simulink model "building_EXAMPLE_v1"  (R2016b)
settings: Solver=ode23tb  StartTime=-building.preruntime+8760*3600  StopTime=building.runtime+8760*3600  MaxStep=600  EnableMultiTasking=on
StartFcn:
  | tic
StopFcn:
  | toc
values from neighbouring files (symbols this model uses):
  building = create_building_automatic(building, modify, import_mode, name_XML, name_EXCEL, name_PHPP, NUMBEROFZONES)    [work_EXAMPLE_v1.m]
undefined symbols (not defined in the file or in its folder): A, B, C, cp, Dd, Dreifach, FluidMix, get_building, ID, MassFlow, p, Pressure, Qdot_C, Qdot_C_energy, Qdot_H, Qdot_H_energy, Qdot_I_electricity, Qdot_I_electricity_energy, Qdot_I_light, Qdot_I_light_energy, Qdot_I_person, Qdot_I_person_energy, Qdot_S, Qdot_S_energy, Qdot_T_ground, Qdot_T_ground_energy, Qdot_T_neighbour, Qdot_T_neighbour_energy, Qdot_T_opaque, Qdot_T_opaque_energy, Qdot_T_window, Qdot_T_window_energy, Qdot_V_infiltration, Qdot_V_infiltration_energy, Qdot_V_mech, Qdot_V_mech_energy, Qdot_V_window, Qdot_V_window_energy, rho, Tc, Temperature, Tr, Ts, Wärmeschutzglas, x_CO2, x_H2O, x_VOC
libraries: carnotUIBK x1931, carnot x83, simulink_extras x22, simulink x12
(part 3 of 35)

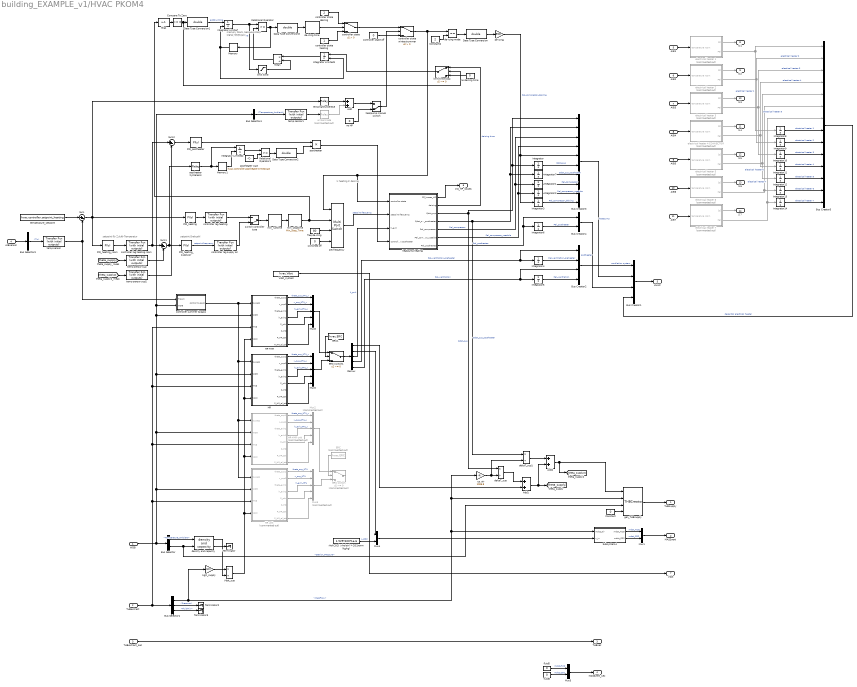
== system building_EXAMPLE_v1/HVAC PKOM4 ==
  note: setpoint Drehzahl
  note: setpoint für Zuluft-Temperatur
  note: memory block,
      | because sharp
      | signal necessary
  note: 1: heating
      | 2: deicing
  WDB : Inport
  THBextract : Inport  Port=2
  THBextract_sec : Inport  Port=3
  AIBsensor : Inport  Port=4
  AIB1 : Inport  Port=5
  AIB2 : Inport  Port=6
  AIB3 : Inport  Port=7
  AIB4 : Inport  Port=8
  AIB5 : Inport  Port=9
  AIB6 : Inport  Port=10
  AIB7 : Inport  Port=11
  Add : Sum
  Add1 : Sum
  Add2 : Sum
  Bias : Bias  Bias=-1
  Bus Creator1 : BusCreator  Inputs=4
  Bus Creator2 : BusCreator  Inputs=4
  Bus Creator3 : BusCreator  Inputs=10
  Bus Creator4 : BusCreator  Inputs=2
  Bus Creator5 : BusCreator  Inputs=14
  Bus Selector : BusSelector  OutputSignals=Temperature_Ambient,Station_Pressure
  Bus Selector1 : BusSelector  OutputSignals=MassFlow,Pressure,FluidMix
  Bus Selector3 : BusSelector  OutputSignals=Ts
  Bus Selector4 : BusSelector  OutputSignals=Temperature_Ambient
  Compare To Zero : simulink/Logic and Bit Operations/Compare To Zero  relop=>=  OutDataTypeStr=uint8
  Constant : Constant  Value=0
  Constant2 : Constant  Value=2
  Data Type Conversion{,1..3} (4 alike) : DataTypeConversion  OutDataTypeStr=double
  Demux : Demux  Outputs=5
  ERC : Constant  Commented=on  Value=hvac.ERC
  ERC switch : Switch  Commented=on  Criteria=u2 ~= 0
  ERC switch1 : Switch  Criteria=u2 ~= 0
  ERC1 : Constant  Value=hvac.ERC
  Einschalthysterese : Relay  OnSwitchValue=0.5  OffSwitchValue=-0.5
  HR : Subsystem  mask{p_el=hvac.HRC_NTU_lu.p_el, low_lim=hvac.HRC_NTU_lu.preheater, Vdot=hvac.HRC_NTU_lu.Vdot, NTU=hvac.HRC_NTU_lu.NTU, NTU_x=hvac.HRC_NTU_lu.NTU_x, vent_sup=off, vent_ext=on, vent_amb=on, vent_exh=off}
      mask prompts: p_el "specific ventilator power in [Wh/m^3]"; low_lim "ambient temperature at which pre-heater starts"; Vdot "volume flow in [m^3/h] for NTU"; NTU_x "NTU of moisture recovery"; vent_sup "ventilator in supply air"; vent_ext "ventilator in extract air"; vent_amb "ventilator in ambient air"; vent_exh "ventilator in exhaust air"
  HR unit : Subsystem  Commented=on  mask{theta_amb2=hvac.HRC_NTU(hvac.system).theta_amb, theta_ext1=hvac.HRC_NTU(hvac.system).theta_ext, Vdot=hvac.HRC_NTU(hvac.system).Vdot, P_el=hvac.HRC_NTU(hvac.system).p_el, rec=hvac.HRC_NTU(hvac.system).eta_phi, low_lim=hvac.HRC_NTU(hvac.system).preheater, vent_sup=off, vent_exh=off, vent_amb=on, vent_ext=on}
      mask prompts: theta_amb2 "ambient air temperature for NTU calculation"; theta_ext1 "extract air temperature for NTU calculation"; Vdot "volume flow in [m^3/h] for NTU"; P_el "specific ventilator power in [Wh/m^3]"; rec "efficiency of heat recovery (by PHI)"; low_lim "ambient temperature at which pre-heater starts"; vent_sup "ventilator in supply air"; vent_exh "ventilator in exhaust air"; vent_amb "ventilator in ambient air"; vent_ext "ventilator in extract air"
      mask init:
      | cp_a = heat_capacity(theta_ext1,1E5,2,0);
      | rho_a = density(theta_ext1,1E5,2,0);
      | mdot_cp = Vdot * cp_a * rho_a / 3600;
      | 
      | %%% NTU %%
      | % not humidity (condensation) considered
      | P_elec = P_el * Vdot;
      | 
      | theta_amb1 = theta_amb2;
      | theta_amb0 = theta_amb1 + vent_amb * P_elec/mdot_cp/2;
      | theta_ext0 = theta_ext1 + vent_ext * P_elec/mdot_cp/2;
      | theta_exh1 = theta_ext1 + P_elec/mdot_cp - rec * (theta_ext1 - theta_amb1);
      | theta_exh0 = theta_exh1 - vent_exh * P_elec/mdot_cp/2;
      | theta_sup0 = theta_amb0 + theta_ext0 - theta_exh0;
      | theta_sup1 = theta_sup0 + vent_sup * P_elec/mdot_cp/2;
      | 
      | dtheta_log = (theta_exh0-theta_amb0 + theta_ext0-theta_sup0)/2;
      | 
      | P_HX = mdot_cp * (theta_sup0-theta_amb1);
      | UA = P_HX / dtheta_log;
      | NTU = UA / mdot_cp;
      | 
      | disp(['  NTU = ' num2str(NTU)])
  HR+MR : Subsystem  mask{p_el=hvac.ERC_NTU_lu.p_el, low_lim=hvac.ERC_NTU_lu.preheater, Vdot=hvac.ERC_NTU_lu.Vdot, NTU=hvac.ERC_NTU_lu.NTU, NTU_x=hvac.ERC_NTU_lu.NTU_x, vent_sup=off, vent_ext=on, vent_amb=on, vent_exh=off}
      mask prompts: p_el "specific ventilator power in [Wh/m^3]"; low_lim "ambient temperature at which pre-heater starts"; Vdot "volume flow in [m^3/h] for NTU"; NTU_x "NTU of moisture recovery"; vent_sup "ventilator in supply air"; vent_ext "ventilator in extract air"; vent_amb "ventilator in ambient air"; vent_exh "ventilator in exhaust air"
  HR+MR unit : Subsystem  Commented=on  mask{theta_amb2=hvac.ERC_NTU(hvac.system).theta_amb, theta_ext1=hvac.ERC_NTU(hvac.system).theta_ext, Vdot=hvac.ERC_NTU(hvac.system).Vdot, P_el=hvac.ERC_NTU(hvac.system).p_el, rec=hvac.ERC_NTU(hvac.system).eta_phi, low_lim=hvac.ERC_NTU(hvac.system).preheater, NTU_x=hvac.ERC_NTU(hvac.system).NTU_x, vent_sup=off, vent_exh=off, vent_amb=on, vent_ext=on}
      mask prompts: theta_amb2 "ambient air temperature for NTU calculation"; theta_ext1 "extract air temperature for NTU calculation"; Vdot "volume flow in [m^3/h] for NTU"; P_el "specific ventilator power in [Wh/m^3]"; rec "efficiency of heat recovery (by PHI)"; low_lim "ambient temperature at which pre-heater starts"; NTU_x "NTU of moisture recovery"; vent_sup "ventilator in supply air"; vent_exh "ventilator in exhaust air"; vent_amb "ventilator in ambient air"; vent_ext "ventilator in extract air"
      mask init:
      | cp_a = heat_capacity(theta_ext1,1E5,2,0);
      | rho_a = density(theta_ext1,1E5,2,0);
      | mdot_cp = Vdot * cp_a * rho_a / 3600;
      | 
      | %%% NTU %%
      | % not humidity (condensation) considered
      | P_elec = P_el * Vdot;
      | 
      | theta_amb1 = theta_amb2;
      | theta_amb0 = theta_amb1 + vent_amb * P_elec/mdot_cp/2;
      | theta_ext0 = theta_ext1 + vent_ext * P_elec/mdot_cp/2;
      | theta_exh1 = theta_ext1 + P_elec/mdot_cp - rec * (theta_ext1 - theta_amb1);
      | theta_exh0 = theta_exh1 - vent_exh * P_elec/mdot_cp/2;
      | theta_sup0 = theta_amb0 + theta_ext0 - theta_exh0;
      | theta_sup1 = theta_sup0 + vent_sup * P_elec/mdot_cp/2;
      | 
      | dtheta_log = (theta_exh0-theta_amb0 + theta_ext0-theta_sup0)/2;
      | 
      | P_HX = mdot_cp * (theta_sup0-theta_amb1);
      | UA = P_HX / dtheta_log;
      | NTU = UA / mdot_cp;
      | 
      | disp(['  NTU = ' num2str(NTU)])
      | disp(['  NTU_x = ' num2str(NTU_x)])
  Integrator{,1..14} (15 alike) : Integrator
  Integrator Limited : Integrator  ExternalReset=rising  LimitOutput=on  LowerSaturationLimit=0
  Integrator Limited1 : Integrator  ExternalReset=rising  LimitOutput=on  LowerSaturationLimit=0
  Integrator Limited2 : Integrator  ExternalReset=either  LimitOutput=on  LowerSaturationLimit=0
  Memory : Memory
  Memory1 : Memory
  Mux1 : Mux  Inputs=2
  Mux2 : Mux  Commented=on  Inputs=5
  Mux3 : Mux  Inputs=2
  Mux4 : Mux  Inputs=2
  Mux5 : Mux  Commented=on  Inputs=5
  Mux6 : Mux  Inputs=5
  Mux8 : Mux  Inputs=5
  PID_heating : simulink/Continuous/PID Controller  Controller=PI  TimeDomain=Continuous-time  SampleTime=-1  IntegratorMethod=Forward Euler  FilterMethod=Forward Euler  Form=Ideal  UseFilter=on  ControllerParametersSource=internal  P=2  I=0.01  D=0  N=100  InitialConditionSource=internal  InitialConditionForIntegrator=0  InitialConditionForFilter=0  ExternalReset=none  LimitOutput=on  UpperSaturationLimit=80  LowerSaturationLimit=0  LinearizeAsGain=on  AntiWindupMode=clamping  Kb=1  TrackingMode=off  Kt=1  PParamMin=[]  PParamMax=[]  IParamMin=[]  IParamMax=[]  DParamMin=[]  DParamMax=[]  NParamMin=[]  NParamMax=[]  KbParamMin=[]  KbParamMax=[]  KtParamMin=[]  KtParamMax=[]  POutMin=[]  POutMax=[]  IOutMin=[]  IOutMax=[]  DOutMin=[]  DOutMax=[]  NOutMin=[]  NOutMax=[]  KbOutMin=[]  KbOutMax=[]  KtOutMin=[]  KtOutMax=[]  IntegratorOutMin=[]  IntegratorOutMax=[]  FilterOutMin=[]  FilterOutMax=[]  SumOutMin=[]  SumOutMax=[]  SumI1OutMin=[]  SumI1OutMax=[]  SumI2OutMin=[]  SumI2OutMax=[]  SumI3OutMin=[]  SumI3OutMax=[]  SumDOutMin=[]  SumDOutMax=[]  SaturationOutMin=[]  SaturationOutMax=[]  IntegratorContinuousStateAttributes=''  IntegratorStateMustResolveToSignalObject=off  IntegratorRTWStateStorageClass=Auto  FilterContinuousStateAttributes=''  FilterStateMustResolveToSignalObject=off  FilterRTWStateStorageClass=Auto  DifferentiatorICPrevScaledInput=0  DifferentiatorOutMin=[]  DifferentiatorOutMax=[]
  PID_heating_room : simulink/Continuous/PID Controller  Controller=PI  TimeDomain=Continuous-time  SampleTime=-1  IntegratorMethod=Forward Euler  FilterMethod=Forward Euler  Form=Ideal  UseFilter=on  ControllerParametersSource=internal  P=hvac.controller.PID_heating_room.P  I=hvac.controller.PID_heating_room.I  D=0  N=100  InitialConditionSource=internal  InitialConditionForIntegrator=0  InitialConditionForFilter=0  ExternalReset=none  LimitOutput=on  UpperSaturationLimit=hvac.controller.PID_heating_room.upper_limit  LowerSaturationLimit=hvac.controller.PID_heating_room.lower_limit  LinearizeAsGain=on  AntiWindupMode=clamping  Kb=1  TrackingMode=off  Kt=1  PParamMin=[]  PParamMax=[]  IParamMin=[]  IParamMax=[]  DParamMin=[]  DParamMax=[]  NParamMin=[]  NParamMax=[]  KbParamMin=[]  KbParamMax=[]  KtParamMin=[]  KtParamMax=[]  POutMin=[]  POutMax=[]  IOutMin=[]  IOutMax=[]  DOutMin=[]  DOutMax=[]  NOutMin=[]  NOutMax=[]  KbOutMin=[]  KbOutMax=[]  KtOutMin=[]  KtOutMax=[]  IntegratorOutMin=[]  IntegratorOutMax=[]  FilterOutMin=[]  FilterOutMax=[]  SumOutMin=[]  SumOutMax=[]  SumI1OutMin=[]  SumI1OutMax=[]  SumI2OutMin=[]  SumI2OutMax=[]  SumI3OutMin=[]  SumI3OutMax=[]  SumDOutMin=[]  SumDOutMax=[]  SaturationOutMin=[]  SaturationOutMax=[]  IntegratorContinuousStateAttributes=''  IntegratorStateMustResolveToSignalObject=off  IntegratorRTWStateStorageClass=Auto  FilterContinuousStateAttributes=''  FilterStateMustResolveToSignalObject=off  FilterRTWStateStorageClass=Auto  DifferentiatorICPrevScaledInput=0  DifferentiatorOutMin=[]  DifferentiatorOutMax=[]
  PID_heating_supplyair : simulink/Continuous/PID Controller  Controller=PI  TimeDomain=Continuous-time  SampleTime=-1  IntegratorMethod=Forward Euler  FilterMethod=Forward Euler  Form=Ideal  UseFilter=on  ControllerParametersSource=internal  P=hvac.controller.PID_heating_supplyair.P  I=hvac.controller.PID_heating_supplyair.I  D=0  N=100  InitialConditionSource=internal  InitialConditionForIntegrator=0  InitialConditionForFilter=0  ExternalReset=none  LimitOutput=on  UpperSaturationLimit=hvac.controller.PID_heating_supplyair.upper_limit  LowerSaturationLimit=hvac.controller.PID_heating_supplyair.lower_limit  LinearizeAsGain=on  AntiWindupMode=clamping  Kb=1  TrackingMode=off  Kt=1  PParamMin=[]  PParamMax=[]  IParamMin=[]  IParamMax=[]  DParamMin=[]  DParamMax=[]  NParamMin=[]  NParamMax=[]  KbParamMin=[]  KbParamMax=[]  KtParamMin=[]  KtParamMax=[]  POutMin=[]  POutMax=[]  IOutMin=[]  IOutMax=[]  DOutMin=[]  DOutMax=[]  NOutMin=[]  NOutMax=[]  KbOutMin=[]  KbOutMax=[]  KtOutMin=[]  KtOutMax=[]  IntegratorOutMin=[]  IntegratorOutMax=[]  FilterOutMin=[]  FilterOutMax=[]  SumOutMin=[]  SumOutMax=[]  SumI1OutMin=[]  SumI1OutMax=[]  SumI2OutMin=[]  SumI2OutMax=[]  SumI3OutMin=[]  SumI3OutMax=[]  SumDOutMin=[]  SumDOutMax=[]  SaturationOutMin=[]  SaturationOutMax=[]  IntegratorContinuousStateAttributes=''  IntegratorStateMustResolveToSignalObject=off  IntegratorRTWStateStorageClass=Auto  FilterContinuousStateAttributes=''  FilterStateMustResolveToSignalObject=off  FilterRTWStateStorageClass=Auto  DifferentiatorICPrevScaledInput=0  DifferentiatorOutMin=[]  DifferentiatorOutMax=[]
  PID_postheater : simulink/Continuous/PID Controller  Controller=PI  TimeDomain=Continuous-time  SampleTime=-1  IntegratorMethod=Forward Euler  FilterMethod=Forward Euler  Form=Ideal  UseFilter=on  ControllerParametersSource=internal  P=hvac.controller.postheater.PID.P  I=hvac.controller.postheater.PID.I  D=0  N=100  InitialConditionSource=internal  InitialConditionForIntegrator=0  InitialConditionForFilter=0  ExternalReset=none  LimitOutput=on  UpperSaturationLimit=hvac.controller.postheater.PID.upper_limit  LowerSaturationLimit=hvac.controller.postheater.PID.lower_limit  LinearizeAsGain=on  AntiWindupMode=clamping  Kb=1  TrackingMode=off  Kt=1  PParamMin=[]  PParamMax=[]  IParamMin=[]  IParamMax=[]  DParamMin=[]  DParamMax=[]  NParamMin=[]  NParamMax=[]  KbParamMin=[]  KbParamMax=[]  KtParamMin=[]  KtParamMax=[]  POutMin=[]  POutMax=[]  IOutMin=[]  IOutMax=[]  DOutMin=[]  DOutMax=[]  NOutMin=[]  NOutMax=[]  KbOutMin=[]  KbOutMax=[]  KtOutMin=[]  KtOutMax=[]  IntegratorOutMin=[]  IntegratorOutMax=[]  FilterOutMin=[]  FilterOutMax=[]  SumOutMin=[]  SumOutMax=[]  SumI1OutMin=[]  SumI1OutMax=[]  SumI2OutMin=[]  SumI2OutMax=[]  SumI3OutMin=[]  SumI3OutMax=[]  SumDOutMin=[]  SumDOutMax=[]  SaturationOutMin=[]  SaturationOutMax=[]  IntegratorContinuousStateAttributes=''  IntegratorStateMustResolveToSignalObject=off  IntegratorRTWStateStorageClass=Auto  FilterContinuousStateAttributes=''  FilterStateMustResolveToSignalObject=off  FilterRTWStateStorageClass=Auto  DifferentiatorICPrevScaledInput=0  DifferentiatorOutMin=[]  DifferentiatorOutMax=[]
  Relational Operator : RelationalOperator  OutDataTypeStr=boolean  RndMeth=Simplest
  Relational Operator1 : RelationalOperator  OutDataTypeStr=boolean  RndMeth=Simplest
  Subsystem4 : Subsystem
  Sum : Sum  Inputs=|+-
  Sum1 : Sum  Inputs=|+-
  Sum2 : Sum  Inputs=|+-
  Terminator : Terminator
  Terminator2 : Terminator
  Terminator3 : Terminator
  Vdot_sup : Product  Inputs=*/
  Vdot_system : Constant  Value=hvac.Vdot
  controller lag heating : simulink_extras/Additional Linear/Transfer Fcn (with initial outputs)  N=[1]  D=[60 1]  Y0=20  U0=0
  controller lag heating room : simulink_extras/Additional Linear/Transfer Fcn (with initial outputs)  N=[1]  D=[60 1]  Y0=20  U0=0
  controller lag supply air : simulink_extras/Additional Linear/Transfer Fcn (with initial outputs)  N=[1]  D=[60 1]  Y0=20  U0=0
  controller state : Switch  Criteria=u2 > Threshold
  controller state deicing : Constant  Value=2
  controller state heating : Constant
  controller state off : Constant  Value=0
  controller state winter/summer : Switch  Criteria=u2 > Threshold
  controller summer bypass : Subsystem
  cp_air : Gain  Gain=1006.8
  de-icing : Gain  Gain=550
  de-icing mode : RelationalOperator  Operator===  OutDataTypeStr=boolean  RndMeth=Simplest
  de-icing time : carnot/Control/Min_Run_Time  tminrun=hvac.controller.deicing_time  mv=1
  deltaT_sup : Product  Inputs=*/
  deltaT_sup1 : Product  Inputs=*/
  density and capacity : carnotUIBK/general/density and capacity
  electrical heater 1 : Subsystem  Commented=on  mask{theta_r_t=hvac.controller.electricalheater.zone(1).theta_r_t, theta_r_t_low=hvac.controller.electricalheater.zone(1).theta_r_t_low, max_power=hvac.controller.electricalheater.zone(1).max_power, part_rad=hvac.controller.electricalheater.zone(1).part_rad, timeconstant_heater=hvac.controller.electricalheater.zone(1).timeconstant_heater, Kp=hvac.controller.electricalheater.zone(1).Kp, Tn=hvac.controller.electricalheater.zone(1).Tn, control_time_values=hvac.controller.electricalheater.zone(1).control_time_values, control_time_duration=hvac.controller.electricalheater.zone(1).control_time_duration, control_time_output=hvac.controller.electricalheater.zone(1).control_time_output}
      mask prompts: theta_r_t "setpoint"; theta_r_t_low "setpoint off/night"; max_power "maximal power"; part_rad "part of radiation"; timeconstant_heater "timeconstant heater"; Kp "PID Kp"; Tn "PID Tn"; control_time_values "control time values"; control_time_duration "control time duration"; control_time_output "control time output"
  electrical heater 2 : Subsystem  Commented=on  mask{theta_r_t=hvac.controller.electricalheater.zone(2).theta_r_t, theta_r_t_low=hvac.controller.electricalheater.zone(2).theta_r_t_low, max_power=hvac.controller.electricalheater.zone(2).max_power, part_rad=hvac.controller.electricalheater.zone(2).part_rad, timeconstant_heater=hvac.controller.electricalheater.zone(2).timeconstant_heater, Kp=hvac.controller.electricalheater.zone(2).Kp, Tn=hvac.controller.electricalheater.zone(2).Tn, control_time_values=hvac.controller.electricalheater.zone(2).control_time_values, control_time_duration=hvac.controller.electricalheater.zone(2).control_time_duration, control_time_output=hvac.controller.electricalheater.zone(2).control_time_output}
      mask prompts: theta_r_t "setpoint"; theta_r_t_low "setpoint off/night"; max_power "maximal power"; part_rad "part of radiation"; timeconstant_heater "timeconstant heater"; Kp "PID Kp"; Tn "PID Tn"; control_time_values "control time values"; control_time_duration "control time duration"; control_time_output "control time output"
  electrical heater 3 : Subsystem  Commented=on  mask{theta_r_t=hvac.controller.electricalheater.zone(3).theta_r_t, theta_r_t_low=hvac.controller.electricalheater.zone(3).theta_r_t_low, max_power=hvac.controller.electricalheater.zone(3).max_power, part_rad=hvac.controller.electricalheater.zone(3).part_rad, timeconstant_heater=hvac.controller.electricalheater.zone(3).timeconstant_heater, Kp=hvac.controller.electricalheater.zone(3).Kp, Tn=hvac.controller.electricalheater.zone(3).Tn, control_time_values=hvac.controller.electricalheater.zone(3).control_time_values, control_time_duration=hvac.controller.electricalheater.zone(3).control_time_duration, control_time_output=hvac.controller.electricalheater.zone(3).control_time_output}
      mask prompts: theta_r_t "setpoint"; theta_r_t_low "setpoint off/night"; max_power "maximal power"; part_rad "part of radiation"; timeconstant_heater "timeconstant heater"; Kp "PID Kp"; Tn "PID Tn"; control_time_values "control time values"; control_time_duration "control time duration"; control_time_output "control time output"
  electrical heater 4 CONVECTOR : Subsystem  Commented=on  mask{theta_r_t=hvac.controller.electricalheater.zone(4).theta_r_t, theta_r_t_low=hvac.controller.electricalheater.zone(4).theta_r_t_low, max_power=hvac.controller.electricalheater.zone(4).max_power, part_rad=hvac.controller.electricalheater.zone(4).part_rad, timeconstant_heater=hvac.controller.electricalheater.zone(4).timeconstant_heater, Kp=hvac.controller.electricalheater.zone(4).Kp, Tn=hvac.controller.electricalheater.zone(4).Tn, control_time_values=hvac.controller.electricalheater.zone(4).control_time_values, control_time_duration=hvac.controller.electricalheater.zone(4).control_time_duration, control_time_output=hvac.controller.electricalheater.zone(4).control_time_output}
      mask prompts: theta_r_t "setpoint"; theta_r_t_low "setpoint off/night"; max_power "maximal power"; part_rad "part of radiation"; timeconstant_heater "timeconstant heater"; Kp "PID Kp"; Tn "PID Tn"; control_time_values "control time values"; control_time_duration "control time duration"; control_time_output "control time output"
  electrical heater 5 : Subsystem  Commented=on  mask{theta_r_t=hvac.controller.electricalheater.zone(5).theta_r_t, theta_r_t_low=hvac.controller.electricalheater.zone(5).theta_r_t_low, max_power=hvac.controller.electricalheater.zone(5).max_power, part_rad=hvac.controller.electricalheater.zone(5).part_rad, timeconstant_heater=hvac.controller.electricalheater.zone(5).timeconstant_heater, Kp=hvac.controller.electricalheater.zone(5).Kp, Tn=hvac.controller.electricalheater.zone(5).Tn, control_time_values=hvac.controller.electricalheater.zone(5).control_time_values, control_time_duration=hvac.controller.electricalheater.zone(5).control_time_duration, control_time_output=hvac.controller.electricalheater.zone(5).control_time_output}
      mask prompts: theta_r_t "setpoint"; theta_r_t_low "setpoint off/night"; max_power "maximal power"; part_rad "part of radiation"; timeconstant_heater "timeconstant heater"; Kp "PID Kp"; Tn "PID Tn"; control_time_values "control time values"; control_time_duration "control time duration"; control_time_output "control time output"
  electrical heater 6 : Subsystem  Commented=on  mask{theta_r_t=hvac.controller.electricalheater.zone(6).theta_r_t, theta_r_t_low=hvac.controller.electricalheater.zone(6).theta_r_t_low, max_power=hvac.controller.electricalheater.zone(6).max_power, part_rad=hvac.controller.electricalheater.zone(6).part_rad, timeconstant_heater=hvac.controller.electricalheater.zone(6).timeconstant_heater, Kp=hvac.controller.electricalheater.zone(6).Kp, Tn=hvac.controller.electricalheater.zone(6).Tn, control_time_values=hvac.controller.electricalheater.zone(6).control_time_values, control_time_duration=hvac.controller.electricalheater.zone(6).control_time_duration, control_time_output=hvac.controller.electricalheater.zone(6).control_time_output}
      mask prompts: theta_r_t "setpoint"; theta_r_t_low "setpoint off/night"; max_power "maximal power"; part_rad "part of radiation"; timeconstant_heater "timeconstant heater"; Kp "PID Kp"; Tn "PID Tn"; control_time_values "control time values"; control_time_duration "control time duration"; control_time_output "control time output"
  electrical heater 7 : Subsystem  Commented=on  mask{theta_r_t=hvac.controller.electricalheater.zone(7).theta_r_t, theta_r_t_low=hvac.controller.electricalheater.zone(7).theta_r_t_low, max_power=hvac.controller.electricalheater.zone(7).max_power, part_rad=hvac.controller.electricalheater.zone(7).part_rad, timeconstant_heater=hvac.controller.electricalheater.zone(7).timeconstant_heater, Kp=hvac.controller.electricalheater.zone(7).Kp, Tn=hvac.controller.electricalheater.zone(7).Tn, control_time_values=hvac.controller.electricalheater.zone(7).control_time_values, control_time_duration=hvac.controller.electricalheater.zone(7).control_time_duration, control_time_output=hvac.controller.electricalheater.zone(7).control_time_output}
      mask prompts: theta_r_t "setpoint"; theta_r_t_low "setpoint off/night"; max_power "maximal power"; part_rad "part of radiation"; timeconstant_heater "timeconstant heater"; Kp "PID Kp"; Tn "PID Tn"; control_time_values "control time values"; control_time_duration "control time duration"; control_time_output "control time output"
  fluid5 : Constant  Value=0
  fluid6 : Constant  Value=0
  freq de-icing : Constant  Value=80
  gen_THBsupply : carnot/Basic/Hydraulics/THBCreator  Inport_ID=off  Inport_T=on  Inport_mdot=on  Inport_p=on  Inport_type=off  Inport_mix=on  Inport_d=off  Inport_c=off  Inport_l=off  Inport_q=off  Inport_LH=off  Inport_H=off  ID=20001  T=20  mdot=0  p=1e5  FluidType=2  FluidMix=0  d=0.125  c=0  l=0  q=0  LH=0  H=0  Annotation_ID=off  Annotation_T=off  Annotation_mdot=off  Annotation_p=off  Annotation_type=off  Annotation_mix=off  Annotation_d=off  Annotation_c=off  Annotation_l=off  Annotation_q=off  Annotation_LH=off  Annotation_H=off
  heatpump heating : Subsystem  mask{heatpump=hvac.HP_ERC}
  heatpump manual switch : ManualSwitch  CurrentSetting=0
  kg/h_supply : Gain  Gain=3600
  limit time : Saturate  UpperLimit=inf  LowerLimit=1
  limit time stop : Switch  Criteria=u2 ~= 0
  mean : Product  Inputs=*/
  min_runtime : carnot/Control/Min_Run_Time  tminrun=hvac.controller.min_runtime  mv=hvac.controller.min_runtime_outputvalue
  min_stoptime : carnot/Control/Min_Stop_Time  tminstop=hvac.controller.min_stoptime
  no HP : Constant  Value=0
  no deicing time : Constant  Value=0
  postheater : Product
  postheater hysteresis : Relay  OnSwitchValue=hvac.controller.postheater.on  OffSwitchValue=hvac.controller.postheater.off
  postheater wait : Constant  Value=hvac.controller.postheater.time2wait
  rho(CO2) / rho(air) * CO2norm (kg/kg) : Constant  Value=1.529*400*1e-6
  set frequency : MultiPortSwitch  Inputs=2  DataPortForDefault=Additional data port  DiagnosticForDefault=None
  switch controller type : ManualSwitch  CurrentSetting=0
  switched off : Constant  Value=0
  temp sensor : simulink_extras/Additional Linear/Transfer Fcn (with initial outputs)  N=[1]  D=[hvac.controller.timeconstant_sensor 1]  Y0=20  U0=0
  temp sensor sup : simulink_extras/Additional Linear/Transfer Fcn (with initial outputs)  N=[1]  D=[hvac.controller.timeconstant_sensor 1]  Y0=20  U0=0
  temp sensor sup2 : simulink_extras/Additional Linear/Transfer Fcn (with initial outputs)  N=[1]  D=[hvac.controller.timeconstant_sensor 1]  Y0=20  U0=0
  temp sensor1 : simulink_extras/Additional Linear/Transfer Fcn (with initial outputs)  N=[1]  D=[hvac.controller.wintermode.amb_temp_timeconstant 1]  Y0=0  U0=0
  temperature_setpoint : Constant  Value=hvac.controller.setpoint_heating
  wintermode : Relay  Commented=on  OnSwitchValue=hvac.controller.wintermode.setpoint_amb_temp+hvac.controller.wintermode.setpoint_amb_temp_hyst  OffSwitchValue=hvac.controller.wintermode.setpoint_amb_temp  OnOutputValue=0  OffOutputValue=1
  THBsupply : Outport
  MASSvent : Outport  Port=2
  THBsec : Outport  Port=3
  MASSvent_sec : Outport  Port=4
  HVAC : Outport  Port=5
  "[S]_HP_losses" : Outport  Port=6
  Vdot : Outport  Port=7
  S 1 : Outport  Port=8
  S 2 : Outport  Port=9
  S 3 : Outport  Port=10
  S 4 : Outport  Port=11
  S 5 : Outport  Port=12
  S 6 : Outport  Port=13
  S 7 : Outport  Port=14
  wires:
  THBextract_sec/1 -> THBsec/1
  Mux3/1 -> MASSvent_sec/1
  fluid5/1 -> Mux3/1  "mdot_H2O"
  fluid6/1 -> Mux3/2  "mdot_CO2"
  Bus Selector/1 -> density and capacity/1  "<Temperature_Ambient>"
  Bus Selector/2 -> gen_THBsupply/3, density and capacity/2  "<Station_Pressure>"
  rho(CO2) / rho(air) * CO2norm (kg/kg)/1 -> Mux4/2  "x_CO2"
  Mux4/1 -> Subsystem4/2(x_in)
  Subsystem4/1(mdot_H2O) -> Mux1/1  "mdot_H2O"
  Subsystem4/2(mdot_CO2) -> Mux1/2  "mdot_CO2"
  Mux1/1 -> MASSvent/1
  Bus Selector1/1 -> cp_air/1, gen_THBsupply/2, Subsystem4/1(mdot_air), kg/h_supply/1  "<MassFlow>"
  density and capacity/1 -> Vdot_sup/2
  density and capacity/2 -> Terminator/1
  gen_THBsupply/1 -> THBsupply/1
  THBextract/1 -> Bus Selector1/1, HR/3(THB), HR+MR/3(THB), HR+MR unit/3(THB), HR unit/3(THB)
  AIBsensor/1 -> Bus Selector3/1
  Bus Creator1/1 -> HVAC/1
  kg/h_supply/1 -> Vdot_sup/1
  Vdot_sup/1 -> HR/4(Vdot), HR+MR/4(Vdot), HR+MR unit/4(Vdot), HR unit/4(Vdot)
  Constant/1 -> gen_THBsupply/4
  Add1/1 -> Add2/2, [theta_supply]
  deltaT_sup/1 -> Add1/1
  temperature_setpoint/1 -> Sum/1
  Bus Selector3/1 -> temp sensor/1  "<Ts>"
  temp sensor/1 -> controller summer bypass/1(Troom), Sum/2
  heatpump heating/3(Qdot_sup) -> deltaT_sup/1, Bus Creator3/1, Integrator/1  "Qdot_sup"
  set frequency/1 -> heatpump heating/2(setpoint frequency)  "setpoint frequency"
  heatpump heating/5(Pel_compressor) -> Bus Creator3/3, Integrator1/1  "Pel_compressor"
  heatpump heating/6(Pel_compressor_useable) -> Bus Creator3/4, Integrator2/1  "Pel_compressor_useable"
  switched off/1 -> set frequency/4
  controller state winter/summer/1 -> set frequency/1, heatpump heating/1(controller state), de-icing mode/1
  freq de-icing/1 -> set frequency/3
  min_runtime/1 -> min_stoptime/1
  min_stoptime/1 -> Bias/1, set frequency/2
  Compare To Zero/1 -> limit time stop/2, Data Type Conversion1/1
  Bias/1 -> Compare To Zero/1
  heatpump heating/2(deicing) -> limit time stop/1  "deicing time"
  Relational Operator/1 -> Data Type Conversion3/1, Memory/1
  controller state heating/1 -> controller state/3
  controller state deicing/1 -> controller state/1
  Constant2/1 -> de-icing mode/2
  de-icing mode/1 -> Data Type Conversion/1
  Data Type Conversion1/1 -> Integrator Limited/1  "add2runtime"
  Data Type Conversion/1 -> de-icing/1
  Integrator Limited/1 -> limit time/1, Relational Operator/1  "actual runtime"
  de-icing time/1 -> controller state/2
  Data Type Conversion3/1 -> de-icing time/1
  Memory/1 -> Integrator Limited/2, Integrator Limited1/2
  Integrator/1 -> Bus Creator3/6  "Qdot_sup"
  Integrator1/1 -> Bus Creator3/8  "Pel_compressor"
  Integrator2/1 -> Bus Creator3/9  "Pel_compressor_useable"
  Integrator3/1 -> Bus Creator3/10  "Pel_compressor_deicing"
  de-icing/1 -> Integrator3/1, Bus Creator3/5  "Pel_compressor_deicing"
  heatpump heating/1("[S]_losses_HP") -> "[S]_HP_losses"/1
  controller state/1 -> controller state winter/summer/1
  controller state off/1 -> controller state winter/summer/3
  Bus Selector1/2 -> Terminator2/1  "<Pressure>"
  Bus Selector1/3 -> Terminator3/1  "<FluidMix>"
  Demux/3 -> heatpump heating/3(h_exh)  "h_exh"
  HR+MR unit/1(theta_sup1) -> Mux2/1  "theta_sup_NTU_x"
  HR+MR unit/2(x_sup1) -> Mux2/2  "x_sup_NTU_x"
  HR+MR unit/4(h_exh1) -> Mux2/3  "h_exh_NTU_x"
  HR unit/1(theta_sup1) -> Mux5/1  "theta_sup_NTU"
  HR unit/2(x_sup1) -> Mux5/2  "x_sup_NTU"
  HR unit/4(h_exh1) -> Mux5/3  "h_exh_NTU"
  Mux5/1 -> ERC switch/3
  Mux2/1 -> ERC switch/1
  Demux/1 -> Add1/2
  Demux/2 -> Mux4/1
  Demux/4 -> Integrator4/1, Bus Creator2/1  "Pel_ventilation_preheater"
  Integrator4/1 -> Bus Creator2/2  "Pel_ventilation_preheater"
  HR+MR unit/5(P_prh) -> Mux2/4
  HR unit/5(P_prh) -> Mux5/4
  HR+MR unit/8(P_HR_el_tot) -> Mux2/5
  HR unit/8(P_HR_el_tot) -> Mux5/5
  Integrator5/1 -> Bus Creator2/4  "Pel_ventilation"
  Demux/5 -> Bus Creator2/3, Integrator5/1  "Pel_ventilation"
  ERC/1 -> ERC switch/2
  controller summer bypass/1(control bypass) -> HR/1(bypass), HR+MR unit/1(bypass), HR unit/1(bypass), HR+MR/1(bypass)
  Vdot_system/1 -> Vdot/1
  Sum1/1 -> postheater hysteresis/1, PID_heating_supplyair/1
  [theta_supply] -> temp sensor sup/1
  PID_heating_room/1 -> controller lag heating room/1
  switch controller type/1 -> min_runtime/1
  PID_heating_supplyair/1 -> controller lag supply air/1  "setpoint frequency"
  PID_heating/1 -> controller lag heating/1
  temp sensor sup/1 -> Sum1/2
  controller lag supply air/1 -> switch controller type/2
  controller lag heating/1 -> switch controller type/1
  mean/1 -> Relational Operator/2
  limit time/1 -> mean/2
  Integrator Limited1/1 -> mean/1
  limit time stop/1 -> Integrator Limited1/1
  no deicing time/1 -> limit time stop/3
  HR+MR/1(theta_sup1) -> Mux8/1  "theta_sup_NTU_x"
  HR+MR/2(x_sup1) -> Mux8/2  "x_sup_NTU_x"
  HR+MR/4(h_exh1) -> Mux8/3  "h_exh_NTU_x"
  HR+MR/5(P_prh) -> Mux8/4
  HR+MR/8(P_HR_el_tot) -> Mux8/5
  controller lag heating room/1 -> Sum2/1, Sum1/1
  Integrator6/1 -> Bus Creator4/2  "Pel_postheater"
  heatpump heating/7(Pel_postheater) -> Integrator6/1, Bus Creator4/1  "Pel_postheater"
  Integrator7/1 -> Bus Creator3/7  "Qdot_sup_postheater"
  heatpump heating/4(Qdot_sup_postheater) -> deltaT_sup1/1, Bus Creator3/2, Integrator7/1  "Qdot_sup_postheater"
  deltaT_sup1/1 -> Add2/1
  cp_air/1 -> deltaT_sup1/2, deltaT_sup/2
  Add2/1 -> [theta_supply2], gen_THBsupply/1
  [theta_supply2] -> temp sensor sup2/1
  temp sensor sup2/1 -> Sum2/2
  postheater hysteresis/1 -> Memory1/1, Integrator Limited2/1
  Sum2/1 -> PID_postheater/1
  Integrator Limited2/1 -> Relational Operator1/1
  postheater/1 -> heatpump heating/4(controller postheater)
  postheater wait/1 -> Relational Operator1/2
  Memory1/1 -> Integrator Limited2/2
  Relational Operator1/1 -> Data Type Conversion2/1
  Data Type Conversion2/1 -> postheater/2
  PID_postheater/1 -> postheater/1
  heatpump manual switch/1 -> controller state winter/summer/2
  ERC1/1 -> ERC switch1/2
  ERC switch1/1 -> Demux/1
  Mux8/1 -> ERC switch1/1
  HR/1(theta_sup1) -> Mux6/1  "theta_sup_NTU_x"
  HR/2(x_sup1) -> Mux6/2  "x_sup_NTU_x"
  HR/4(h_exh1) -> Mux6/3  "h_exh_NTU_x"
  HR/5(P_prh) -> Mux6/4
  HR/8(P_HR_el_tot) -> Mux6/5
  Mux6/1 -> ERC switch1/3
  Sum/1 -> PID_heating/1, Einschalthysterese/1, PID_heating_room/1
  Bus Selector4/1 -> temp sensor1/1  "<Temperature_Ambient>"
  WDB/1 -> Bus Selector/1, HR/2(WDB), HR+MR/2(WDB), Bus Selector4/1, controller summer bypass/2(WDB), HR+MR unit/2(WDB), HR unit/2(WDB)
  temp sensor1/1 -> wintermode/1
  Einschalthysterese/1 -> Add/1
  wintermode/1 -> Add/2
  Add/1 -> heatpump manual switch/1
  no HP/1 -> heatpump manual switch/2
  AIB4/1 -> electrical heater 4 CONVECTOR/1(temperature room)
  electrical heater 4 CONVECTOR/1("[S]") -> S 4/1
  electrical heater 4 CONVECTOR/2(Pel) -> Bus Creator5/4, Integrator11/1  "electrical heater 4"
  electrical heater 7/1("[S]") -> S 7/1
  electrical heater 6/1("[S]") -> S 6/1
  electrical heater 5/1("[S]") -> S 5/1
  electrical heater 3/1("[S]") -> S 3/1
  electrical heater 2/1("[S]") -> S 2/1
  electrical heater 1/1("[S]") -> S 1/1
  AIB5/1 -> electrical heater 5/1(temperature room)
  AIB6/1 -> electrical heater 6/1(temperature room)
  AIB7/1 -> electrical heater 7/1(temperature room)
  AIB3/1 -> electrical heater 3/1(temperature room)
  AIB2/1 -> electrical heater 2/1(temperature room)
  AIB1/1 -> electrical heater 1/1(temperature room)
  electrical heater 3/2(Pel) -> Bus Creator5/3, Integrator10/1  "electrical heater 3"
  electrical heater 2/2(Pel) -> Bus Creator5/2, Integrator9/1  "electrical heater 2"
  electrical heater 1/2(Pel) -> Integrator8/1, Bus Creator5/1  "electrical heater 1"
  electrical heater 5/2(Pel) -> Bus Creator5/5, Integrator12/1  "electrical heater 5"
  electrical heater 6/2(Pel) -> Bus Creator5/6, Integrator13/1  "electrical heater 6"
  electrical heater 7/2(Pel) -> Integrator14/1, Bus Creator5/7  "electrical heater 7"
  Bus Creator2/1 -> Bus Creator1/1  "ventilation system"
  Bus Creator3/1 -> Bus Creator1/2  "heatpump"
  Bus Creator4/1 -> Bus Creator1/3  "postheater"
  Integrator8/1 -> Bus Creator5/8  "electrical heater 1"
  Integrator10/1 -> Bus Creator5/10  "electrical heater 3"
  Integrator9/1 -> Bus Creator5/9  "electrical heater 2"
  Integrator11/1 -> Bus Creator5/11  "electrical heater 4"
  Integrator12/1 -> Bus Creator5/12  "electrical heater 5"
  Integrator13/1 -> Bus Creator5/13  "electrical heater 6"
  Integrator14/1 -> Bus Creator5/14  "electrical heater 7"
  Bus Creator5/1 -> Bus Creator1/4  "decentral electrical heater"

== system building_EXAMPLE_v1/HVAC door opening ==
  profile opening door zone_1 : carnot/Load/General/Repeating_Profile  period=hvac.door_1.timevalues(end)  rep_seq_t=hvac.door_1.timevalues(1:end-1)  rep_seq_d=hvac.door_1.timeduration  rep_seq_y=hvac.door_1.values
  profile opening door zone_2 : carnot/Load/General/Repeating_Profile  period=hvac.door_2.timevalues(end)  rep_seq_t=hvac.door_2.timevalues(1:end-1)  rep_seq_d=hvac.door_2.timeduration  rep_seq_y=hvac.door_2.values
  profile opening door zone_3 : carnot/Load/General/Repeating_Profile  period=hvac.door_3.timevalues(end)  rep_seq_t=hvac.door_3.timevalues(1:end-1)  rep_seq_d=hvac.door_3.timeduration  rep_seq_y=hvac.door_3.values
  profile opening door zone_4 : carnot/Load/General/Repeating_Profile  period=hvac.door_4.timevalues(end)  rep_seq_t=hvac.door_4.timevalues(1:end-1)  rep_seq_d=hvac.door_4.timeduration  rep_seq_y=hvac.door_4.values
  profile opening door zone_5 : carnot/Load/General/Repeating_Profile  period=hvac.door_5.timevalues(end)  rep_seq_t=hvac.door_5.timevalues(1:end-1)  rep_seq_d=hvac.door_5.timeduration  rep_seq_y=hvac.door_5.values
  profile opening door zone_6 : carnot/Load/General/Repeating_Profile  period=hvac.door_6.timevalues(end)  rep_seq_t=hvac.door_6.timevalues(1:end-1)  rep_seq_d=hvac.door_6.timeduration  rep_seq_y=hvac.door_6.values
  op_door1 : Outport
  op_door2 : Outport  Port=2
  op_door3 : Outport  Port=3
  op_door4 : Outport  Port=4
  op_door5 : Outport  Port=5
  op_door6 : Outport  Port=6
  wires:
  profile opening door zone_1/1 -> op_door1/1
  profile opening door zone_2/1 -> op_door2/1
  profile opening door zone_4/1 -> op_door4/1
  profile opening door zone_5/1 -> op_door5/1
  profile opening door zone_6/1 -> op_door6/1
  profile opening door zone_3/1 -> op_door3/1

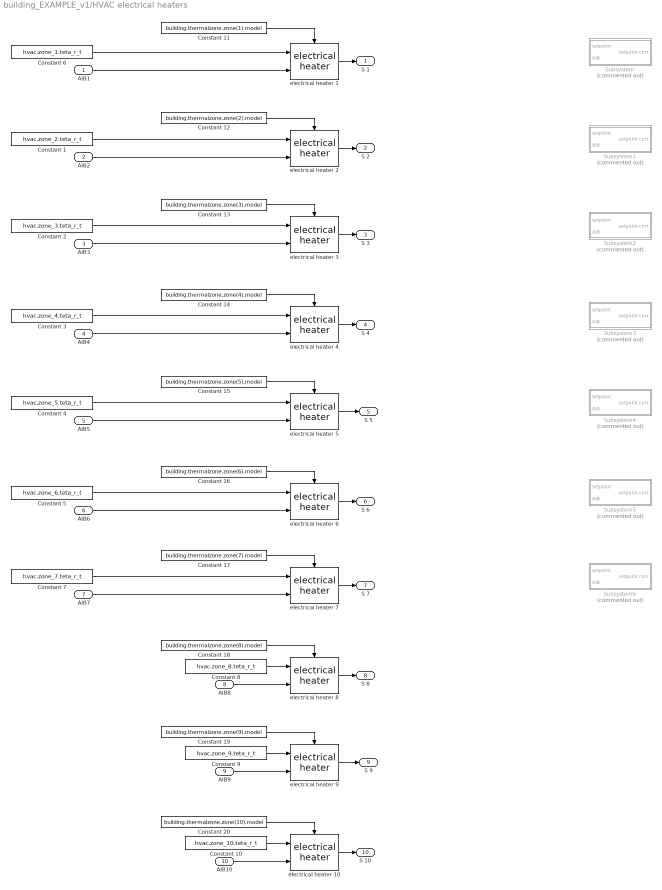
== system building_EXAMPLE_v1/HVAC electrical heaters ==
  AIB1 : Inport
  AIB2 : Inport  Port=2
  AIB3 : Inport  Port=3
  AIB4 : Inport  Port=4
  AIB5 : Inport  Port=5
  AIB6 : Inport  Port=6
  AIB7 : Inport  Port=7
  AIB8 : Inport  Port=8
  AIB9 : Inport  Port=9
  AIB10 : Inport  Port=10
  Constant 1 : Constant  Value=hvac.zone_2.teta_r_t  VectorParams1D=off
  Constant 10 : Constant  Value=hvac.zone_10.teta_r_t  VectorParams1D=off
  Constant 11 : Constant  Value=building.thermalzone.zone(1).model  VectorParams1D=off
  Constant 12 : Constant  Value=building.thermalzone.zone(2).model  VectorParams1D=off
  Constant 13 : Constant  Value=building.thermalzone.zone(3).model  VectorParams1D=off
  Constant 14 : Constant  Value=building.thermalzone.zone(4).model  VectorParams1D=off
  Constant 15 : Constant  Value=building.thermalzone.zone(5).model  VectorParams1D=off
  Constant 16 : Constant  Value=building.thermalzone.zone(6).model  VectorParams1D=off
  Constant 17 : Constant  Value=building.thermalzone.zone(7).model  VectorParams1D=off
  Constant 18 : Constant  Value=building.thermalzone.zone(8).model  VectorParams1D=off
  Constant 19 : Constant  Value=building.thermalzone.zone(9).model  VectorParams1D=off
  Constant 2 : Constant  Value=hvac.zone_3.teta_r_t  VectorParams1D=off
  Constant 20 : Constant  Value=building.thermalzone.zone(10).model  VectorParams1D=off
  Constant 3 : Constant  Value=hvac.zone_4.teta_r_t  VectorParams1D=off
  Constant 4 : Constant  Value=hvac.zone_5.teta_r_t  VectorParams1D=off
  Constant 5 : Constant  Value=hvac.zone_6.teta_r_t  VectorParams1D=off
  Constant 6 : Constant  Value=hvac.zone_1.teta_r_t  VectorParams1D=off
  Constant 7 : Constant  Value=hvac.zone_7.teta_r_t  VectorParams1D=off
  Constant 8 : Constant  Value=hvac.zone_8.teta_r_t  VectorParams1D=off
  Constant 9 : Constant  Value=hvac.zone_9.teta_r_t  VectorParams1D=off
  Subsystem : Subsystem  Commented=on
  Subsystem1 : Subsystem  Commented=on
  Subsystem2 : Subsystem  Commented=on
  Subsystem3 : Subsystem  Commented=on
  Subsystem4 : Subsystem  Commented=on
  Subsystem5 : Subsystem  Commented=on
  Subsystem6 : Subsystem  Commented=on
  electrical heater 1 : carnotUIBK/HVAC/electrical heater  max_power=hvac.zone_1.max_power
  electrical heater 10 : carnotUIBK/HVAC/electrical heater  max_power=hvac.zone_10.max_power
  electrical heater 2 : carnotUIBK/HVAC/electrical heater  max_power=hvac.zone_2.max_power
  electrical heater 3 : carnotUIBK/HVAC/electrical heater  max_power=hvac.zone_3.max_power
  electrical heater 4 : carnotUIBK/HVAC/electrical heater  max_power=hvac.zone_4.max_power
  electrical heater 5 : carnotUIBK/HVAC/electrical heater  max_power=hvac.zone_5.max_power
  electrical heater 6 : carnotUIBK/HVAC/electrical heater  max_power=hvac.zone_6.max_power
  electrical heater 7 : carnotUIBK/HVAC/electrical heater  max_power=hvac.zone_7.max_power
  electrical heater 8 : carnotUIBK/HVAC/electrical heater  max_power=hvac.zone_8.max_power
  electrical heater 9 : carnotUIBK/HVAC/electrical heater  max_power=hvac.zone_9.max_power
  S 1 : Outport
  S 2 : Outport  Port=2
  S 3 : Outport  Port=3
  S 4 : Outport  Port=4
  S 5 : Outport  Port=5
  S 6 : Outport  Port=6
  S 7 : Outport  Port=7
  S 8 : Outport  Port=8
  S 9 : Outport  Port=9
  S 10 : Outport  Port=10
  wires:
  AIB1/1 -> electrical heater 1/2
  electrical heater 1/1 -> S 1/1
  Constant 11/1 -> electrical heater 1/Enable
  electrical heater 2/1 -> S 2/1
  AIB2/1 -> electrical heater 2/2
  AIB3/1 -> electrical heater 3/2
  electrical heater 3/1 -> S 3/1
  AIB4/1 -> electrical heater 4/2
  electrical heater 4/1 -> S 4/1
  electrical heater 5/1 -> S 5/1
  electrical heater 6/1 -> S 6/1
  AIB7/1 -> electrical heater 7/2
  electrical heater 7/1 -> S 7/1
  AIB8/1 -> electrical heater 8/2
  electrical heater 8/1 -> S 8/1
  AIB9/1 -> electrical heater 9/2
  electrical heater 9/1 -> S 9/1
  AIB10/1 -> electrical heater 10/2
  electrical heater 10/1 -> S 10/1
  Constant 7/1 -> electrical heater 7/1
  Constant 8/1 -> electrical heater 8/1
  Constant 9/1 -> electrical heater 9/1
  Constant 10/1 -> electrical heater 10/1
  Constant 12/1 -> electrical heater 2/Enable
  Constant 13/1 -> electrical heater 3/Enable
  Constant 14/1 -> electrical heater 4/Enable
  Constant 15/1 -> electrical heater 5/Enable
  Constant 16/1 -> electrical heater 6/Enable
  Constant 17/1 -> electrical heater 7/Enable
  Constant 18/1 -> electrical heater 8/Enable
  Constant 19/1 -> electrical heater 9/Enable
  Constant 20/1 -> electrical heater 10/Enable
  Constant 6/1 -> electrical heater 1/1
  Constant 2/1 -> electrical heater 3/1
  Constant 1/1 -> electrical heater 2/1
  Constant 4/1 -> electrical heater 5/1
  Constant 5/1 -> electrical heater 6/1
  Constant 3/1 -> electrical heater 4/1
  AIB5/1 -> electrical heater 5/2
  AIB6/1 -> electrical heater 6/2
